simulink model "PubIfDecisionPLAN_MDL_DS"  (R2020b)
settings: configuration reference "DspaceConfig" (kept outside this file)
PostLoadFcn:
  | if any(exist('dsrtsu_mdlpostloadfcn', 'file') ~= 0), dsrtsu_mdlpostloadfcn('Execute', bdroot); end
InitFcn:
  | , if any(exist('rtifpga_mdlclblib', 'file') ~= 0), rtifpga_mdlclblib('Init', bdroot); end,
  | , if any(exist('dsmpb_private', 'file') ~= 0), dsmpb_private('dsmpb_mdlclblib', 'Init', bdroot); end,
libraries: simulink x7
PreSaveFcn:
  | , if any(exist('dsmpb_private', 'file') ~= 0), dsmpb_private('dsmpb_mdlclblib', 'PreSave', bdroot); end,
CloseFcn:
  | , if any(exist('dsmpb_private', 'file') ~= 0), dsmpb_private('dsmpb_mdlclblib', 'Close', bdroot); end,
settings Model: DataDictionary=PLAN_all.sldd  RTICANMMDATA=struct('GeneralSetupData',struct('modelroot','C:\Users\GW00133806\Desktop\ADAS_Store\Project\V61_Autobox_Noa_Nofusion','generalsettings',struct('filesettings',struct('destfolder',struct('Name','RTICANMM_FILES','Check',1),'buildfolder',struct('Name','.','Check',1),'AbsDestfolder',struct('Name','C:\Users\GW00133806\Desktop\ADAS_Store\Project\V61_Autobox_Noa_Nofusion\RTICANMM_FILES'),'AbsBuildfolder',struct('Name','C:\Users\GW00133806\Desktop\ADAS_Store\Project\V61_Autobox_Noa_Nofusion'))),'options',struct('addpaths',1,'rmpaths',1,'addtrcexclusion',false,'cannavigator',struct('checkmonitoring',0),'show_usrtrc',0,'use_usrtrc',0),'advanced',struct('options',ones(1,100)),'MPSetup',{{}},'RTI',struct('Type','DSRT','Ver','4.4','Date','02-Nov-2020'),'modelname','PubIfDecisionPLAN_MDL_DS','block','PubIfDecisionPLAN_MDL_DS'))  DSRTSU_INTERNAL_RTIFPGA=170  OrderedModelArguments=off  Creator=GW00180895  LastModifiedBy=GW00133806
settings ConfigSetRef: SourceName=DspaceConfig

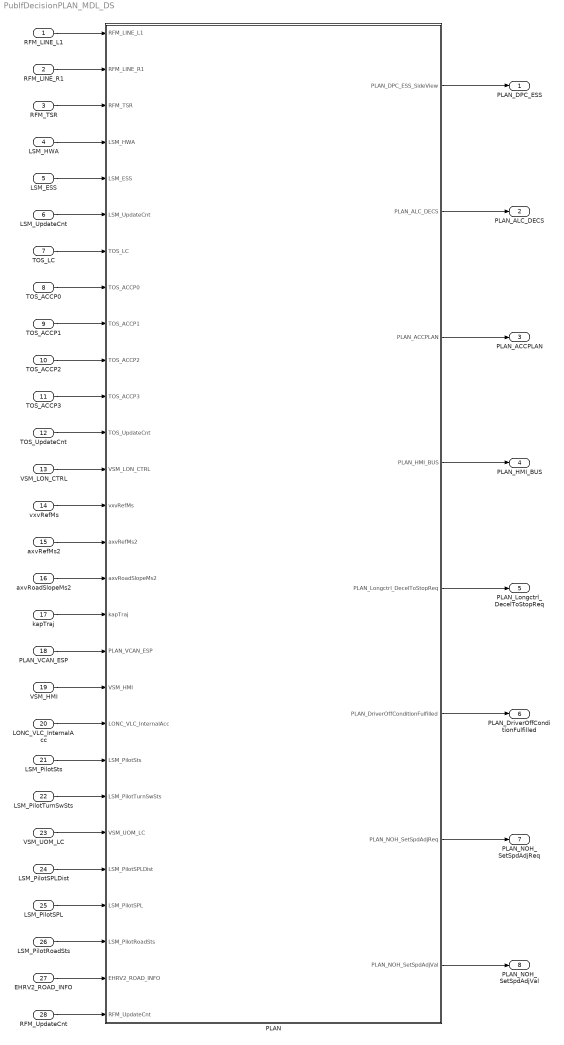
== system PubIfDecisionPLAN_MDL_DS ==
  RFM_LINE_L1 : Inport  OutDataTypeStr=Bus: RFM_LINE_BUS  PortDimensions=1  BusOutputAsStruct=on
  RFM_LINE_R1 : Inport  Port=2  OutDataTypeStr=Bus: RFM_LINE_BUS  PortDimensions=1  BusOutputAsStruct=on
  RFM_TSR : Inport  Port=3  OutDataTypeStr=Bus: RFM_TSR_BUS  PortDimensions=1  BusOutputAsStruct=on
  LSM_HWA : Inport  Port=4  OutDataTypeStr=Bus: LSM_HWA_BUS  PortDimensions=1  BusOutputAsStruct=on
  LSM_ESS : Inport  Port=5  OutDataTypeStr=Bus: LSM_ESS_BUS  PortDimensions=1  BusOutputAsStruct=on
  LSM_UpdateCnt : Inport  Port=6  OutDataTypeStr=uint32  PortDimensions=1  BusOutputAsStruct=on
  TOS_LC : Inport  Port=7  OutDataTypeStr=Bus: TOS_LC_BUS  PortDimensions=1  BusOutputAsStruct=on
  TOS_ACCP0 : Inport  Port=8  OutDataTypeStr=Bus: TOS_ACCP0_BUS  PortDimensions=1  BusOutputAsStruct=on
  TOS_ACCP1 : Inport  Port=9  OutDataTypeStr=Bus: TOS_ACCP1_BUS  PortDimensions=1  BusOutputAsStruct=on
  TOS_ACCP2 : Inport  Port=10  OutDataTypeStr=Bus: TOS_ACCP2_BUS  PortDimensions=1  BusOutputAsStruct=on
  TOS_ACCP3 : Inport  Port=11  OutDataTypeStr=Bus: TOS_ACCP3_BUS  PortDimensions=1  BusOutputAsStruct=on
  TOS_UpdateCnt : Inport  Port=12  OutDataTypeStr=uint32  PortDimensions=1  BusOutputAsStruct=on
  VSM_LON_CTRL : Inport  Port=13  OutDataTypeStr=Bus: VSM_LON_CTRL_BUS  PortDimensions=1  BusOutputAsStruct=on
  vxvRefMs : Inport  Port=14  OutDataTypeStr=single  PortDimensions=1  BusOutputAsStruct=on
  axvRefMs2 : Inport  Port=15  OutDataTypeStr=single  PortDimensions=1  BusOutputAsStruct=on
  axvRoadSlopeMs2 : Inport  Port=16  OutDataTypeStr=single  PortDimensions=1  BusOutputAsStruct=on
  kapTraj : Inport  Port=17  OutDataTypeStr=single  PortDimensions=1  BusOutputAsStruct=on
  PLAN_VCAN_ESP : Inport  Port=18  OutDataTypeStr=Bus: VCAN_ESP_MSG_BUS  PortDimensions=1  BusOutputAsStruct=on
  VSM_HMI : Inport  Port=19  OutDataTypeStr=Bus: VSM_HMI_BUS  PortDimensions=1  BusOutputAsStruct=on
  LONC_VLC_InternalAcc : Inport  Port=20  OutDataTypeStr=single  PortDimensions=1  BusOutputAsStruct=on
  LSM_PilotSts : Inport  Port=21  OutDataTypeStr=uint8  PortDimensions=1  BusOutputAsStruct=on
  LSM_PilotTurnSwSts : Inport  Port=22  OutDataTypeStr=uint8  PortDimensions=1  BusOutputAsStruct=on
  VSM_UOM_LC : Inport  Port=23  OutDataTypeStr=Bus: VSM_UOM_LC_BUS  PortDimensions=1  BusOutputAsStruct=on
  LSM_PilotSPLDist : Inport  Port=24  OutDataTypeStr=uint16
  LSM_PilotSPL : Inport  Port=25  OutDataTypeStr=uint8
  LSM_PilotRoadSts : Inport  Port=26  OutDataTypeStr=uint8
  EHRV2_ROAD_INFO : Inport  Port=27  OutDataTypeStr=Bus: EHRV2_ROAD_INFO_BUS
  RFM_UpdateCnt : Inport  Port=28
  PLAN : Subsystem
  PLAN_DPC_ESS : Outport  OutDataTypeStr=Bus: PLAN_DPC_ESS_BUS  PortDimensions=1  BusOutputAsStruct=on
  PLAN_ALC_DECS : Outport  Port=2  OutDataTypeStr=Bus: PLAN_ALC_DECS_BUS  PortDimensions=1  BusOutputAsStruct=on
  PLAN_ACCPLAN : Outport  Port=3  OutDataTypeStr=Bus: PLAN_ACCPLAN_BUS  PortDimensions=1  BusOutputAsStruct=on
  PLAN_HMI_BUS : Outport  Port=4  OutDataTypeStr=Bus: PLAN_HMI_BUS
  PLAN_Longctrl_DecelToStopReq : Outport  Port=5  OutDataTypeStr=boolean
  PLAN_DriverOffConditionFulfilled : Outport  Port=6  OutDataTypeStr=boolean
  PLAN_NOH_SetSpdAdjReq : Outport  Port=7  OutDataTypeStr=boolean
  PLAN_NOH_SetSpdAdjVal : Outport  Port=8  OutDataTypeStr=uint8
  wires:
  RFM_LINE_L1/1 -> PLAN/1(RFM_LINE_L1)
  RFM_LINE_R1/1 -> PLAN/2(RFM_LINE_R1)
  RFM_TSR/1 -> PLAN/3(RFM_TSR)
  LSM_HWA/1 -> PLAN/4(LSM_HWA)
  LSM_ESS/1 -> PLAN/5(LSM_ESS)
  LSM_UpdateCnt/1 -> PLAN/6(LSM_UpdateCnt)
  TOS_LC/1 -> PLAN/7(TOS_LC)
  TOS_ACCP0/1 -> PLAN/8(TOS_ACCP0)
  TOS_ACCP1/1 -> PLAN/9(TOS_ACCP1)
  TOS_ACCP2/1 -> PLAN/10(TOS_ACCP2)
  TOS_ACCP3/1 -> PLAN/11(TOS_ACCP3)
  TOS_UpdateCnt/1 -> PLAN/12(TOS_UpdateCnt)
  VSM_LON_CTRL/1 -> PLAN/13(VSM_LON_CTRL)
  vxvRefMs/1 -> PLAN/14(vxvRefMs)
  axvRefMs2/1 -> PLAN/15(axvRefMs2)
  axvRoadSlopeMs2/1 -> PLAN/16(axvRoadSlopeMs2)
  kapTraj/1 -> PLAN/17(kapTraj)
  PLAN_VCAN_ESP/1 -> PLAN/18(PLAN_VCAN_ESP)
  VSM_HMI/1 -> PLAN/19(VSM_HMI)
  LSM_PilotSts/1 -> PLAN/21(LSM_PilotSts)
  LSM_PilotTurnSwSts/1 -> PLAN/22(LSM_PilotTurnSwSts)
  VSM_UOM_LC/1 -> PLAN/23(VSM_UOM_LC)
  PLAN/1(PLAN_DPC_ESS_SideView) -> PLAN_DPC_ESS/1
  PLAN/3(PLAN_ACCPLAN) -> PLAN_ACCPLAN/1
  PLAN/2(PLAN_ALC_DECS) -> PLAN_ALC_DECS/1
  LONC_VLC_InternalAcc/1 -> PLAN/20(LONC_VLC_InternalAcc)
  PLAN/4(PLAN_HMI_BUS) -> PLAN_HMI_BUS/1
  PLAN/5(PLAN_Longctrl_DecelToStopReq) -> PLAN_Longctrl_DecelToStopReq/1
  PLAN/6(PLAN_DriverOffConditionFulfilled) -> PLAN_DriverOffConditionFulfilled/1
  LSM_PilotSPLDist/1 -> PLAN/24(LSM_PilotSPLDist)
  LSM_PilotSPL/1 -> PLAN/25(LSM_PilotSPL)
  LSM_PilotRoadSts/1 -> PLAN/26(LSM_PilotRoadSts)
  PLAN/7(PLAN_NOH_SetSpdAdjReq) -> PLAN_NOH_SetSpdAdjReq/1
  PLAN/8(PLAN_NOH_SetSpdAdjVal) -> PLAN_NOH_SetSpdAdjVal/1
  EHRV2_ROAD_INFO/1 -> PLAN/27(EHRV2_ROAD_INFO)
  RFM_UpdateCnt/1 -> PLAN/28(RFM_UpdateCnt)

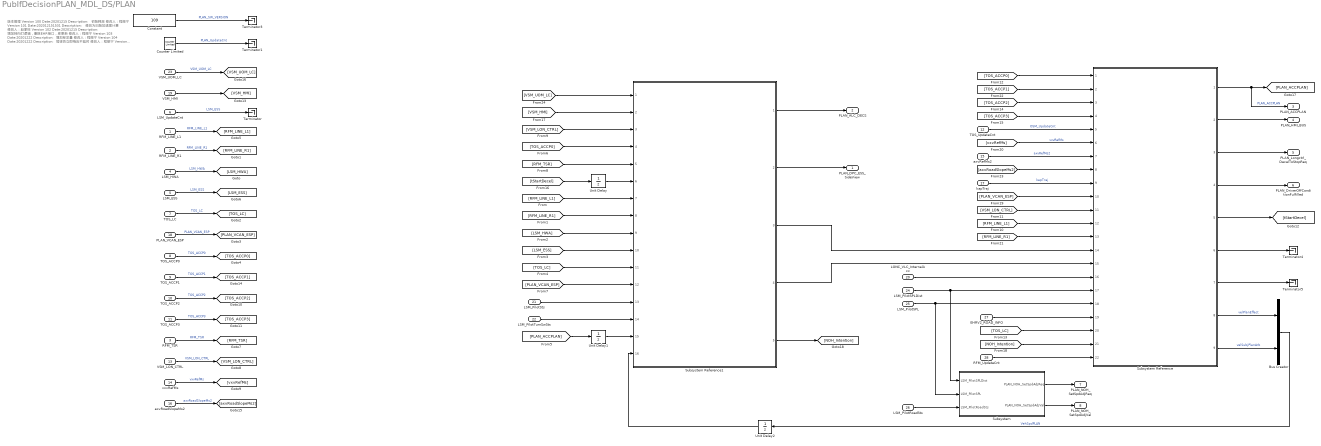
== system PubIfDecisionPLAN_MDL_DS/PLAN ==
  note: 版本管理
      | Version 100
      | Date:20201215
      | Description: 初版释放
      | 修改人：程振宁
      |
      | Version 101
      | Date:202012151531
      | Description: 修改为旧版加速度计算
      | 修改人：赵家旺
      |
      | Version 102
      | Date:20201215
      | Description: 增加转向灯逻辑，删除EHR接口，库更新
      | 修改人：程振宁
      |
      | Version 103
      | Date:20201222
      | Description: 增加标定量
      | 修改人：程振宁
      |
      | Version 104
      | Date:20201222
      | Description: 驾驶员立即响应不延时
      | 修改人：程振宁
      |
      | Version 105
      | Date:20201229
      | Description: 拆分
      | 修改人：程振宁
      |
      | Version 106
      | Date:20210106
      | Description: 接口修改
      | 修改人：程振宁
      |
      | Version 107
      | Date:20210312
      | Description: 根据加塞需求修改AP接口
      | 修改人：赵家旺
      |
      | Version 108
      | Date:20210315
      | Description: PLAN添加EHRV2接口
      | 修改人：赵家旺
      |
      | Version 109
      | Date:20210318
      | Description: PLAN添加RFM_UpdateCnt接口
      | 修改人：赵家旺
  RFM_LINE_L1 : Inport  OutDataTypeStr=Bus: RFM_LINE_BUS  PortDimensions=1  Interpolate=off  BusOutputAsStruct=on
  RFM_LINE_R1 : Inport  Port=2  OutDataTypeStr=Bus: RFM_LINE_BUS  PortDimensions=1  Interpolate=off  BusOutputAsStruct=on
  RFM_TSR : Inport  Port=3  OutDataTypeStr=Bus: RFM_TSR_BUS  PortDimensions=1  Interpolate=off  BusOutputAsStruct=on
  LSM_HWA : Inport  Port=4  OutDataTypeStr=Bus: LSM_HWA_BUS  PortDimensions=1  Interpolate=off  BusOutputAsStruct=on
  LSM_ESS : Inport  Port=5  OutDataTypeStr=Bus: LSM_ESS_BUS  PortDimensions=1  Interpolate=off  BusOutputAsStruct=on
  LSM_UpdateCnt : Inport  Port=6  OutDataTypeStr=uint32  PortDimensions=1  Interpolate=off  BusOutputAsStruct=on
  TOS_LC : Inport  Port=7  OutDataTypeStr=Bus: TOS_LC_BUS  PortDimensions=1  BusOutputAsStruct=on
  TOS_ACCP0 : Inport  Port=8  OutDataTypeStr=Bus: TOS_ACCP0_BUS  PortDimensions=1  BusOutputAsStruct=on
  TOS_ACCP1 : Inport  Port=9  OutDataTypeStr=Bus: TOS_ACCP1_BUS  LockScale=on
  TOS_ACCP2 : Inport  Port=10  OutDataTypeStr=Bus: TOS_ACCP2_BUS
  TOS_ACCP3 : Inport  Port=11  OutDataTypeStr=Bus: TOS_ACCP3_BUS
  TOS_UpdateCnt : Inport  Port=12
  VSM_LON_CTRL : Inport  Port=13  OutDataTypeStr=Bus: VSM_LON_CTRL_BUS  PortDimensions=1  Interpolate=off  BusOutputAsStruct=on
  vxvRefMs : Inport  Port=14  OutDataTypeStr=single  PortDimensions=1  Interpolate=off  BusOutputAsStruct=on
  axvRefMs2 : Inport  Port=15
  axvRoadSlopeMs2 : Inport  Port=16
  kapTraj : Inport  Port=17
  PLAN_VCAN_ESP : Inport  Port=18  OutDataTypeStr=Bus: VCAN_ESP_MSG_BUS
  VSM_HMI : Inport  Port=19  OutDataTypeStr=Bus: VSM_HMI_BUS
  LONC_VLC_InternalAcc : Inport  Port=20  OutDataTypeStr=single
  LSM_PilotSts : Inport  Port=21
  LSM_PilotTurnSwSts : Inport  Port=22
  VSM_UOM_LC : Inport  Port=23  OutDataTypeStr=Bus: VSM_UOM_LC_BUS
  LSM_PilotSPLDist : Inport  Port=24  OutDataTypeStr=uint16
  LSM_PilotSPL : Inport  Port=25  OutDataTypeStr=uint8
  LSM_PilotRoadSts : Inport  Port=26  OutDataTypeStr=uint8
  EHRV2_ROAD_INFO : Inport  Port=27  OutDataTypeStr=Bus: EHRV2_ROAD_INFO_BUS
  RFM_UpdateCnt : Inport  Port=28
  Bus Creator : BusCreator  Inputs=2
  Constant : Constant  Value=109  OutDataTypeStr=uint8
  Counter Limited : simulink/Sources/Counter Limited  uplimit=255  tsamp=-1
  Subsystem : Subsystem
  Subsystem Reference : Subsystem  ReferencedSubsystem=AP
  Subsystem Reference1 : Subsystem  ReferencedSubsystem=PLAN_ALC
  Terminator{,1,3..5} (5 alike) : Terminator
  Unit Delay : UnitDelay  SampleTime=-1  HasFrameUpgradeWarning=on
  Unit Delay1 : UnitDelay  SampleTime=-1  HasFrameUpgradeWarning=on
  Unit Delay2 : UnitDelay  SampleTime=-1  HasFrameUpgradeWarning=on
  PLAN_DPC_ESS_SideView : Outport  OutDataTypeStr=Bus: PLAN_DPC_ESS_BUS
  PLAN_ALC_DECS : Outport  Port=2  OutDataTypeStr=Bus: PLAN_ALC_DECS_BUS
  PLAN_ACCPLAN : Outport  Port=3  OutDataTypeStr=Bus: PLAN_ACCPLAN_BUS
  PLAN_HMI_BUS : Outport  Port=4  OutDataTypeStr=Bus: PLAN_HMI_BUS
  PLAN_Longctrl_DecelToStopReq : Outport  Port=5  OutDataTypeStr=boolean
  PLAN_DriverOffConditionFulfilled : Outport  Port=6  OutDataTypeStr=boolean
  PLAN_NOH_SetSpdAdjReq : Outport  Port=7  OutDataTypeStr=boolean
  PLAN_NOH_SetSpdAdjVal : Outport  Port=8  OutDataTypeStr=uint8
  wires:
  RFM_TSR/1 -> [RFM_TSR]  "RFM_TSR"
  TOS_ACCP3/1 -> [TOS_ACCP3]  "TOS_ACCP3"
  RFM_LINE_L1/1 -> [RFM_LINE_L1]  "RFM_LINE_L1"
  axvRoadSlopeMs2/1 -> [axvRoadSlopeMs2]  "axvRoadSlopeMs2"
  TOS_ACCP0/1 -> [TOS_ACCP0]  "TOS_ACCP0"
  LSM_UpdateCnt/1 -> Terminator/1  "LSM_ESS"
  vxvRefMs/1 -> [vxvRefMs]  "vxvRefMs"
  VSM_HMI/1 -> [VSM_HMI]
  TOS_ACCP2/1 -> [TOS_ACCP2]  "TOS_ACCP2"
  LSM_HWA/1 -> [LSM_HWA]  "LSM_HWA"
  RFM_LINE_R1/1 -> [RFM_LINE_R1]  "RFM_LINE_R1"
  [tStartDecel] -> Unit Delay/1
  VSM_LON_CTRL/1 -> [VSM_LON_CTRL]  "VSM_LON_CTRL"
  LSM_ESS/1 -> [LSM_ESS]  "LSM_ESS"
  PLAN_VCAN_ESP/1 -> [PLAN_VCAN_ESP]  "PLAN_VCAN_ESP"
  Counter Limited/1 -> Terminator1/1  "PLAN_UpdateCnt"
  TOS_ACCP1/1 -> [TOS_ACCP1]  "TOS_ACCP1"
  TOS_LC/1 -> [TOS_LC]  "TOS_LC"
  Constant/1 -> Terminator3/1  "PLAN_SW_VERSION"
  VSM_UOM_LC/1 -> [VSM_UOM_LC]  "VSM_UOM_LC"
  [RFM_LINE_R1] -> Subsystem Reference/13
  TOS_UpdateCnt/1 -> Subsystem Reference/5  "OSM_UpdateCnt"
  [TOS_ACCP0] -> Subsystem Reference/1
  [RFM_LINE_L1] -> Subsystem Reference/12
  [vxvRefMs] -> Subsystem Reference/6  "vxvRefMs"
  [TOS_ACCP2] -> Subsystem Reference/3
  LONC_VLC_InternalAcc/1 -> Subsystem Reference/16
  kapTraj/1 -> Subsystem Reference/9  "kapTraj"
  axvRefMs2/1 -> Subsystem Reference/7  "axvRefMs2"
  [TOS_ACCP3] -> Subsystem Reference/4
  [VSM_LON_CTRL] -> Subsystem Reference/11
  [PLAN_VCAN_ESP] -> Subsystem Reference/10
  Subsystem Reference/1 -> PLAN_ACCPLAN/1, [PLAN_ACCPLAN]  "PLAN_ACCPLAN"
  Subsystem Reference/5 -> [tStartDecel]
  Subsystem Reference1/4 -> Subsystem Reference/15
  Subsystem Reference1/3 -> Subsystem Reference/14
  [TOS_ACCP1] -> Subsystem Reference/2
  [axvRoadSlopeMs2] -> Subsystem Reference/8
  Subsystem Reference/2 -> PLAN_HMI_BUS/1
  Subsystem Reference/3 -> PLAN_Longctrl_DecelToStopReq/1
  Subsystem Reference/4 -> PLAN_DriverOffConditionFulfilled/1
  Subsystem Reference1/1 -> PLAN_ALC_DECS/1
  Subsystem Reference1/2 -> PLAN_DPC_ESS_SideView/1
  LSM_PilotRoadSts/1 -> Subsystem/3(LSM_PilotRoadSts)
  LSM_PilotSPLDist/1 -> Subsystem/1(LSM_PilotSPLDist), Subsystem Reference/17
  LSM_PilotSPL/1 -> Subsystem/2(LSM_PilotSPL), Subsystem Reference/18
  Subsystem Reference/6 -> Terminator4/1
  Subsystem Reference/7 -> Terminator5/1
  Subsystem/1(PLAN_NOH_SetSpdAdjReq) -> PLAN_NOH_SetSpdAdjReq/1
  Subsystem/2(PLAN_NOH_SetSpdAdjVal) -> PLAN_NOH_SetSpdAdjVal/1
  Unit Delay/1 -> Subsystem Reference1/6
  [VSM_LON_CTRL] -> Subsystem Reference1/3
  [PLAN_VCAN_ESP] -> Subsystem Reference1/12
  [TOS_ACCP0] -> Subsystem Reference1/4
  [TOS_LC] -> Subsystem Reference1/11
  [RFM_TSR] -> Subsystem Reference1/5
  [LSM_ESS] -> Subsystem Reference1/10
  [LSM_HWA] -> Subsystem Reference1/9
  [RFM_LINE_R1] -> Subsystem Reference1/8
  [VSM_HMI] -> Subsystem Reference1/2
  [RFM_LINE_L1] -> Subsystem Reference1/7
  [VSM_UOM_LC] -> Subsystem Reference1/1
  LSM_PilotSts/1 -> Subsystem Reference1/13
  LSM_PilotTurnSwSts/1 -> Subsystem Reference1/14
  [PLAN_ACCPLAN] -> Unit Delay1/1
  Unit Delay1/1 -> Subsystem Reference1/15
  Subsystem Reference/8 -> Bus Creator/1  "velPlanEffect"
  Subsystem Reference/9 -> Bus Creator/2  "velSubjPlanArb"
  Bus Creator/1 -> Unit Delay2/1  "VehSpdPLAN"
  Unit Delay2/1 -> Subsystem Reference1/16
  Subsystem Reference1/5 -> [NOH_Intention]
  [TOS_LC] -> Subsystem Reference/20
  [NOH_Intention] -> Subsystem Reference/21
  EHRV2_ROAD_INFO/1 -> Subsystem Reference/19
  RFM_UpdateCnt/1 -> Subsystem Reference/22

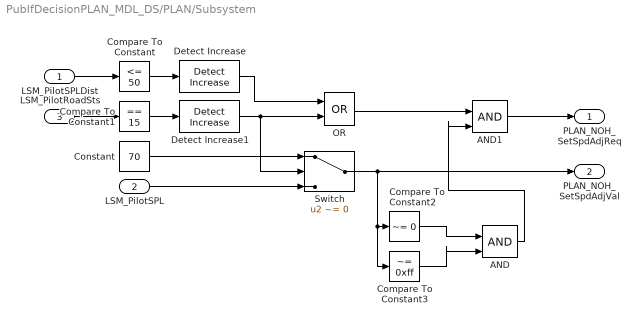
== system PubIfDecisionPLAN_MDL_DS/PLAN/Subsystem ==
  LSM_PilotSPLDist : Inport
  LSM_PilotSPL : Inport  Port=2
  LSM_PilotRoadSts : Inport  Port=3
  AND : Logic  IconShape=distinctive  AllPortsSameDT=off  OutDataTypeStr=boolean
  AND1 : Logic  IconShape=distinctive  AllPortsSameDT=off  OutDataTypeStr=boolean
  Compare To Constant : simulink/Logic and Bit Operations/Compare To Constant  relop=<=  const=50  OutDataTypeStr=boolean
  Compare To Constant1 : simulink/Logic and Bit Operations/Compare To Constant  relop===  const=15  OutDataTypeStr=boolean
  Compare To Constant2 : simulink/Logic and Bit Operations/Compare To Constant  relop=~=  const=0  OutDataTypeStr=boolean
  Compare To Constant3 : simulink/Logic and Bit Operations/Compare To Constant  relop=~=  const=0xff  OutDataTypeStr=boolean
  Constant : Constant  Value=70  OutDataTypeStr=uint8
  Detect Increase : simulink/Logic and Bit Operations/Detect Increase  vinit=0.0  OutDataTypeStr=boolean
  Detect Increase1 : simulink/Logic and Bit Operations/Detect Increase  vinit=0.0  OutDataTypeStr=boolean
  OR : Logic  Operator=OR  AllPortsSameDT=off  OutDataTypeStr=boolean
  Switch : Switch  Criteria=u2 ~= 0
  PLAN_NOH_SetSpdAdjReq : Outport
  PLAN_NOH_SetSpdAdjVal : Outport  Port=2
  wires:
  LSM_PilotSPLDist/1 -> Compare To Constant/1
  Detect Increase/1 -> OR/1
  LSM_PilotSPL/1 -> Switch/3
  LSM_PilotRoadSts/1 -> Compare To Constant1/1
  OR/1 -> AND1/1
  Compare To Constant/1 -> Detect Increase/1
  Detect Increase1/1 -> Switch/2, OR/2
  Compare To Constant1/1 -> Detect Increase1/1
  Switch/1 -> Compare To Constant3/1, Compare To Constant2/1, PLAN_NOH_SetSpdAdjVal/1
  Constant/1 -> Switch/1
  Compare To Constant2/1 -> AND/1
  Compare To Constant3/1 -> AND/2
  AND1/1 -> PLAN_NOH_SetSpdAdjReq/1
  AND/1 -> AND1/2
